simulink model "Offline_DataImport_AND_ECGAnalysis_AND_SCGAnalysis"  (R2020b)
settings: Solver=FixedStepDiscrete  StartTime=0.0  StopTime=param_sim_time  FixedStep=1/fs  MaxStep=1/fs  RelTol=1e-3
undefined symbols (not defined in the file): analyses, fdesignblkfcn, fs, gcbh, param_tot_samples
libraries: dspstat3 x1
(part 3 of 5)

== system Offline_DataImport_AND_ECGAnalysis_AND_SCGAnalysis/ECG Preprocessing/Enabled ECG Preprocessing Subsystem/ECG Filtfiltering/Bandpass Filter 2 ==
  In : Inport
  Generated Filter Block : DiscreteFir  Tag=BlockMethodSubSystem  Coefficients=[-0.0114243088354877773 0.00587624110456374388 0.00413946068324517157 0.00264334557424035672 0.00138774422276622192 0.00039597756815762733 -0.000357391963790950132 -0.000870027328167087902 -0.00118474210009046274 -0.0013114772414377189 -0.00130211118137258525 -0.00117028348293094116 -0.000969555288066135598 -0.000709991739662891794 -0.000441672338585462343 -0.000165596169411169614 7.38618239838010476e-05 0.000289182992126718261 0.00043918297873611449 0.000554539538172022298 0.000596791094711021305 0.000591852861038305242 0.000558642096174625374 0.000449318410474004379 0.000334719809825502479 0.00020575650819831294 5.39363215079843861e-05 -0.000101322531501510382 -0.000240833690149395291 -0.000354646039305753225 -0.000451018706232981029 -0.000523127741752206499 -0.000570171746042747937 -0.000579976289078059509 -0.000560050610609794802 -0.000510203484091005868 -0.000444253999700439106 -0.000361620699264023418 -0.000270418439597897714 -0.000171285996548194847 -6.96491449474114649e-05 2.51074882581126674e-05 0.000107701466472475207 0.000177443554931332875 0.000215288445749358542 0.000245848468855064048 0.000245696970898627229 0.000229649686627229205 0.00019096241212286473 0.000142984412950488554 7.04459950623022302e-05 -8.24128026295257998e-06 -9.80593727097200246e-05 -0.000181512369773678683 -0.000268731962362029828 -0.000342263684306691809 -0.000409113387221587271 -0.000453067377901137172 -0.000486836085121275519 -0.000497275928952340546 -0.00049828288783324709 -0.000472232231767717378 -0.00043821960462679492 -0.000378588991066479766 -0.000316844305738618603 -0.000241178452312015845 -0.000166037327502541535 -8.72939132895780845e-05 -1.92312446675550752e-05 4.72061762121969014e-05 9.32922079647201252e-05 0.000128677828260322091 0.000142225646220916352 0.000145392718308013161 0.000124316294889322346 9.22525950362868691e-05 3.91139366419743922e-05 -2.09540055264127723e-05 -9.84817072707550728e-05 -0.000176447200533612 -0.000261969930569216219 -0.000338398170707415388 -0.000413673787246831778 -0.000474956484152477126 -0.000526126847064748229 -0.000557031780194342657 -0.000573463759814568652 -0.000565518328802135789 -0.000545968260267525388 -0.000503292825521842527 -0.000450686144492560767 -0.00038193732270500047 -0.000310533512604118864 -0.000229221000311531989 -0.000153634622944792687 -7.7008709436998668e-05 -1.29951882972875049e-05 4.41972427699440645e-05 7.97744827227258452e-05 0.000101355022460052069 9.88614688825825011e-05 8.13696224336354218e-05 3.98982051577762009e-05 -1.42484593806998378e-05 -8.82654671942838254e-05 -0.000167074457359766074 -0.00025963077237387 -0.000347989994374806391 -0.000439444994547399936 -0.00051811479354047299 -0.000590082617058047473 -0.000641838802120880611 -0.000681503522967578934 -0.000694804478821137508 -0.00069209853970065606 -0.000663795693677639645 -0.000621757222242421206 -0.000557224399686986893 -0.000484587241980041772 -0.000396687438130890677 -0.000308737174406251494 -0.000214743893139471981 -0.00013218336614707546 -5.38482479860227792e-05 3.99111044497961476e-06 4.92154210607297082e-05 6.74354760492514721e-05 6.74472479585495194e-05 4.02217001782036176e-05 -4.06942016077313506e-06 -7.33562872444193381e-05 -0.000154074998390272069 -0.000252782754343081062 -0.000354062465090758047 -0.000462222943123069205 -0.000562271536985421011 -0.000658661832374597689 -0.000735808311790427799 -0.000799943578584080828 -0.000838241882526128551 -0.000857844739487072239 -0.000847533102258754556 -0.000817418121589637975 -0.000760200301916437102 -0.000687422833072246636 -0.000595027809558780832 -0.000496080524377292761 -0.000387710990138089018 -0.000284208196984854847 -0.000182518571703508756 -9.84384035011120345e-05 -2.73607674165961268e-05 1.77508990696524649e-05 4.21653277528823839e-05 3.53040248291924125e-05 5.59921773045889137e-06 -5.46825757556310132e-05 -0.000133739024050423885 -0.000236066993422962002 -0.000348549704079315764 -0.000473403235651745358 -0.000595572390038458938 -0.000716976323207035166 ...(+20655 chars)]  InputProcessing=Columns as channels (frame based)
  Out : Outport  VectorParamsAs1DForOutWhenUnconnected=off
  wires:
  Generated Filter Block/1 -> Out/1
  In/1 -> Generated Filter Block/1

== system Offline_DataImport_AND_ECGAnalysis_AND_SCGAnalysis/ECG Preprocessing/Enabled ECG Preprocessing Subsystem/To Workspace: Processed ECG/Enabled To Workspace ECG Subsystem ==
  note: The subsystem is only enabled when it receives a (non-zero) signal
  In1 : Inport
  Enable : EnablePort
  To Workspace ECG : ToWorkspace  VariableName=out_ecg_preprocessing  SaveFormat=Structure  SampleTime=-1
  wires:
  In1/1 -> To Workspace ECG/1

== system Offline_DataImport_AND_ECGAnalysis_AND_SCGAnalysis/SCG Analysis/Enabled SCG Analysis Subsystem/Anisotropy Characterization/Average Cycle Max Diameter//Volume Calculator ==
  in_r_pos : Inport
  in_scg_xyz : Inport  Port=2
  S1 Selector : Selector  NumberOfDimensions=2  InputPortWidth=3  IndexOptions=Index vector (dialog),Index vector (dialog)  Indices=[1:fs*0.2],[1 2 3]  OutputSizes=1,1
  SCG xyz Average Cycle : Subsystem
  Wrapped Average Cycle Max Diameter/Volume Calculator : MATLAB Function  TreatAsAtomicUnit=on
  out_average_cycle_max_diameter/volume : Outport
  wires:
  Wrapped Average Cycle Max Diameter/Volume Calculator/1(avg_cycle_max_diameter_over_volume) -> out_average_cycle_max_diameter/volume/1
  SCG xyz Average Cycle/1(out_scg_xyz_avgcycle) -> S1 Selector/1
  in_scg_xyz/1 -> SCG xyz Average Cycle/2(in_scg_xyz)
  in_r_pos/1 -> SCG xyz Average Cycle/1(in_ecg_r)
  S1 Selector/1 -> Wrapped Average Cycle Max Diameter/Volume Calculator/1(avg_s1_xyz)  "avg_scg_xyz_s1"

== system Offline_DataImport_AND_ECGAnalysis_AND_SCGAnalysis/SCG Analysis/Enabled SCG Analysis Subsystem/Anisotropy Characterization/Average Cycle Max//Median Diameter Calculator ==
  in_r_pos : Inport
  in_scg_xyz : Inport  Port=2
  S1 Selector : Selector  NumberOfDimensions=2  InputPortWidth=3  IndexOptions=Index vector (dialog),Index vector (dialog)  Indices=[1:fs*0.2],[1 2 3]  OutputSizes=1,1
  SCG xyz Average Cycle : Subsystem
  Wrapped Average Cycle Max/Median Diameter Calculator : MATLAB Function  TreatAsAtomicUnit=on
  out_average_cycle_max/median_diameter : Outport
  wires:
  Wrapped Average Cycle Max/Median Diameter Calculator/1(avg_cycle_max_over_median_diameter) -> out_average_cycle_max/median_diameter/1
  SCG xyz Average Cycle/1(out_scg_xyz_avgcycle) -> S1 Selector/1
  in_scg_xyz/1 -> SCG xyz Average Cycle/2(in_scg_xyz)
  in_r_pos/1 -> SCG xyz Average Cycle/1(in_ecg_r)
  S1 Selector/1 -> Wrapped Average Cycle Max/Median Diameter Calculator/1(avg_s1_xyz)  "avg_scg_xyz_s1"

== system Offline_DataImport_AND_ECGAnalysis_AND_SCGAnalysis/SCG Analysis/Enabled SCG Analysis Subsystem/Anisotropy Characterization/Average Cycle Max//Min Diameter Calculator ==
  in_r_pos : Inport
  in_scg_xyz : Inport  Port=2
  S1 Selector : Selector  NumberOfDimensions=2  InputPortWidth=3  IndexOptions=Index vector (dialog),Index vector (dialog)  Indices=[1:fs*0.2],[1 2 3]  OutputSizes=1,1
  SCG xyz Average Cycle : Subsystem
  Wrapped Average Cycle Max/Min Diameters Calculator : MATLAB Function  TreatAsAtomicUnit=on
  out_average_cycle_max/min_diameter : Outport
  wires:
  S1 Selector/1 -> Wrapped Average Cycle Max/Min Diameters Calculator/1(avg_s1_xyz)  "avg_scg_xyz_s1"
  in_r_pos/1 -> SCG xyz Average Cycle/1(in_ecg_r)
  in_scg_xyz/1 -> SCG xyz Average Cycle/2(in_scg_xyz)
  SCG xyz Average Cycle/1(out_scg_xyz_avgcycle) -> S1 Selector/1
  Wrapped Average Cycle Max/Min Diameters Calculator/1(avg_cycle_max_over_min_diameters) -> out_average_cycle_max/min_diameter/1

== system Offline_DataImport_AND_ECGAnalysis_AND_SCGAnalysis/SCG Analysis/Enabled SCG Analysis Subsystem/Anisotropy Characterization/Average Max Diameter//Volume Calculator ==
  in_r_pos : Inport
  in_scg_xyz : Inport  Port=2
  Constant1 : Constant  Value=fs
  Wrapped Average Max Diameter/Volume Calculator : MATLAB Function  TreatAsAtomicUnit=on
  out_average_max_diameter/volume : Outport
  wires:
  Constant1/1 -> Wrapped Average Max Diameter/Volume Calculator/1(fs)
  Wrapped Average Max Diameter/Volume Calculator/1(avg_max_diameter_over_volume) -> out_average_max_diameter/volume/1
  in_scg_xyz/1 -> Wrapped Average Max Diameter/Volume Calculator/3(scg_xyz)
  in_r_pos/1 -> Wrapped Average Max Diameter/Volume Calculator/2(r_pos)

== system Offline_DataImport_AND_ECGAnalysis_AND_SCGAnalysis/SCG Analysis/Enabled SCG Analysis Subsystem/Anisotropy Characterization/Average Max//Median Diameter Calculator ==
  in_r_pos : Inport
  in_scg_xyz : Inport  Port=2
  Constant1 : Constant  Value=fs
  Wrapped Average Max/Median Diameter Calculator : MATLAB Function  TreatAsAtomicUnit=on
  out_average_max/median_diameter : Outport
  wires:
  Constant1/1 -> Wrapped Average Max/Median Diameter Calculator/1(fs)
  Wrapped Average Max/Median Diameter Calculator/1(avg_max_over_median_diameter) -> out_average_max/median_diameter/1
  in_scg_xyz/1 -> Wrapped Average Max/Median Diameter Calculator/3(scg_xyz)
  in_r_pos/1 -> Wrapped Average Max/Median Diameter Calculator/2(r_pos)

== system Offline_DataImport_AND_ECGAnalysis_AND_SCGAnalysis/SCG Analysis/Enabled SCG Analysis Subsystem/Anisotropy Characterization/Average Max//Min Diameter Calculator ==
  in_r_pos : Inport
  in_scg_xyz : Inport  Port=2
  Constant1 : Constant  Value=fs
  Wrapped Average Max/Min Diameters Calculator : MATLAB Function  TreatAsAtomicUnit=on
  out_average_max/min_diameter : Outport
  wires:
  in_r_pos/1 -> Wrapped Average Max/Min Diameters Calculator/2(r_pos)
  in_scg_xyz/1 -> Wrapped Average Max/Min Diameters Calculator/3(scg_xyz)
  Wrapped Average Max/Min Diameters Calculator/1(avg_max_over_min_diameters) -> out_average_max/min_diameter/1
  Constant1/1 -> Wrapped Average Max/Min Diameters Calculator/1(fs)

== system Offline_DataImport_AND_ECGAnalysis_AND_SCGAnalysis/SCG Analysis/Enabled SCG Analysis Subsystem/Signal Generation/2D Mod Average Cycle ==
  in_r_pos : Inport
  in_2DMod : Inport  Port=2
  Average 2DMod Cycle Calculator : MATLAB Function  TreatAsAtomicUnit=on
  out_2DMod_avgcycle : Outport  VectorParamsAs1DForOutWhenUnconnected=off
  wires:
  in_r_pos/1 -> Average 2DMod Cycle Calculator/1(r_pos)
  in_2DMod/1 -> Average 2DMod Cycle Calculator/2(signal)
  Average 2DMod Cycle Calculator/1(avg_cycle) -> out_2DMod_avgcycle/1

== system Offline_DataImport_AND_ECGAnalysis_AND_SCGAnalysis/SCG Analysis/Enabled SCG Analysis Subsystem/Signal Generation/2DMod Calculator ==
  in_scg_xyz : Inport
  2DMod Calculator : Subsystem
  Constant : Constant  Value=xyz2Dcombo
  Multiport Switch : MultiPortSwitch
  xy Selector : Selector  NumberOfDimensions=2  IndexOptions=Select all,Index vector (dialog)  Indices=[1:min(analyses.ecg.RR)],[1 2]  OutputSizes=1,1
  xz Selector2 : Selector  NumberOfDimensions=2  IndexOptions=Select all,Index vector (dialog)  Indices=[1:min(analyses.ecg.RR)],[1 3]  OutputSizes=1,1
  yz Selector1 : Selector  NumberOfDimensions=2  IndexOptions=Select all,Index vector (dialog)  Indices=[1:min(analyses.ecg.RR)],[2 3]  OutputSizes=1,1
  out_2DMod : Outport  VectorParamsAs1DForOutWhenUnconnected=off
  wires:
  2DMod Calculator/1(2D Modulus) -> out_2DMod/1
  in_scg_xyz/1 -> xz Selector2/1, xy Selector/1, yz Selector1/1
  Constant/1 -> Multiport Switch/1
  Multiport Switch/1 -> 2DMod Calculator/1(2D Components)
  xy Selector/1 -> Multiport Switch/2
  yz Selector1/1 -> Multiport Switch/3
  xz Selector2/1 -> Multiport Switch/4

== system Offline_DataImport_AND_ECGAnalysis_AND_SCGAnalysis/SCG Analysis/Enabled SCG Analysis Subsystem/Signal Generation/3D Mod Average Cycle ==
  in_r_pos : Inport
  in_3DMod : Inport  Port=2
  Average 3DMod Cycle Calculator : MATLAB Function  TreatAsAtomicUnit=on
  out_3DMod_avgcycle : Outport  VectorParamsAs1DForOutWhenUnconnected=off
  wires:
  Average 3DMod Cycle Calculator/1(avg_cycle) -> out_3DMod_avgcycle/1
  in_3DMod/1 -> Average 3DMod Cycle Calculator/2(signal)
  in_r_pos/1 -> Average 3DMod Cycle Calculator/1(r_pos)

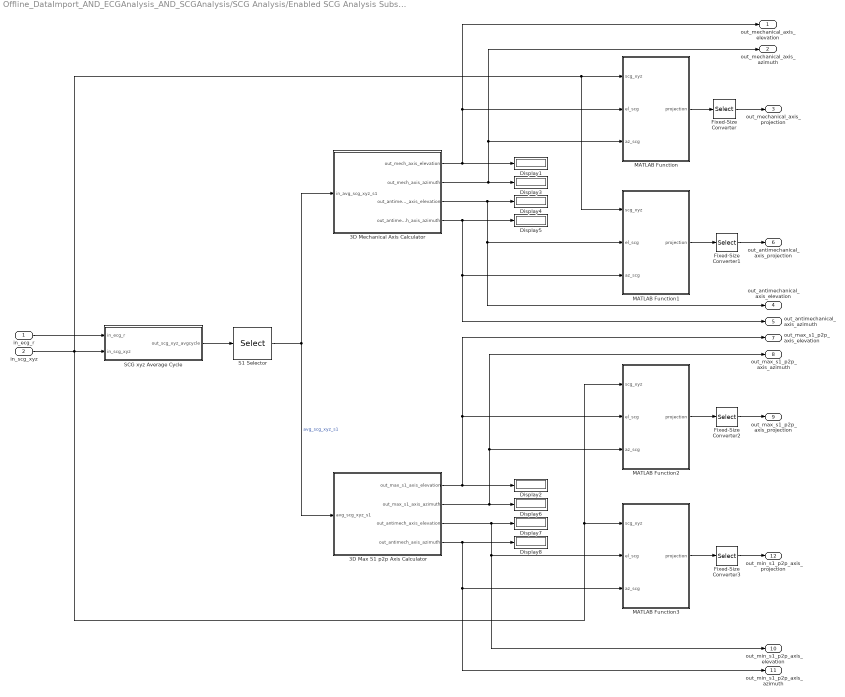
== system Offline_DataImport_AND_ECGAnalysis_AND_SCGAnalysis/SCG Analysis/Enabled SCG Analysis Subsystem/Signal Generation/3D Projections ==
  in_ecg_r : Inport
  in_scg_xyz : Inport  Port=2
  3D Max S1 p2p Axis Calculator : Subsystem
  3D Mechanical Axis Calculator : Subsystem
  Display{1..8} (8 alike) : Display
  Fixed-Size Converter{,1..3} (4 alike) : Selector  NumberOfDimensions=2  IndexOptions=Index vector (dialog),Index vector (dialog)  Indices=[1:param_tot_samples],[1]  OutputSizes=1,1
  MATLAB Function : MATLAB Function  TreatAsAtomicUnit=on
  MATLAB Function1 : MATLAB Function  TreatAsAtomicUnit=on
  MATLAB Function2 : MATLAB Function  TreatAsAtomicUnit=on
  MATLAB Function3 : MATLAB Function  TreatAsAtomicUnit=on
  S1 Selector : Selector  NumberOfDimensions=2  InputPortWidth=3  IndexOptions=Index vector (dialog),Index vector (dialog)  Indices=[1:fs*0.2],[1 2 3]  OutputSizes=1,1
  SCG xyz Average Cycle : Subsystem
  out_mechanical_axis_elevation : Outport
  out_mechanical_axis_azimuth : Outport  Port=2
  out_mechanical_axis_projection : Outport  Port=3
  out_antimechanical_axis_elevation : Outport  Port=4
  out_antimechanical_axis_azimuth : Outport  Port=5
  out_antimechanical_axis_projection : Outport  Port=6
  out_max_s1_p2p_axis_elevation : Outport  Port=7
  out_max_s1_p2p_axis_azimuth : Outport  Port=8
  out_max_s1_p2p_axis_projection : Outport  Port=9
  out_min_s1_p2p_axis_elevation : Outport  Port=10
  out_min_s1_p2p_axis_azimuth : Outport  Port=11
  out_min_s1_p2p_axis_projection : Outport  Port=12
  wires:
  in_scg_xyz/1 -> SCG xyz Average Cycle/2(in_scg_xyz), MATLAB Function/1(scg_xyz), MATLAB Function1/1(scg_xyz), MATLAB Function2/1(scg_xyz), MATLAB Function3/1(scg_xyz)
  S1 Selector/1 -> 3D Max S1 p2p Axis Calculator/1(avg_scg_xyz_s1), 3D Mechanical Axis Calculator/1(in_avg_scg_xyz_s1)  "avg_scg_xyz_s1"
  SCG xyz Average Cycle/1(out_scg_xyz_avgcycle) -> S1 Selector/1
  MATLAB Function2/1(projection) -> Fixed-Size Converter2/1
  MATLAB Function1/1(projection) -> Fixed-Size Converter1/1
  MATLAB Function/1(projection) -> Fixed-Size Converter/1
  Fixed-Size Converter/1 -> out_mechanical_axis_projection/1
  Fixed-Size Converter1/1 -> out_antimechanical_axis_projection/1
  Fixed-Size Converter2/1 -> out_max_s1_p2p_axis_projection/1
  MATLAB Function3/1(projection) -> Fixed-Size Converter3/1
  Fixed-Size Converter3/1 -> out_min_s1_p2p_axis_projection/1
  3D Mechanical Axis Calculator/2(out_mech_axis_azimuth) -> Display3/1, out_mechanical_axis_azimuth/1, MATLAB Function/3(az_scg)
  3D Mechanical Axis Calculator/3(out_antimech_axis_elevation) -> Display4/1, out_antimechanical_axis_elevation/1, MATLAB Function1/2(el_scg)
  3D Mechanical Axis Calculator/1(out_mech_axis_elevation) -> Display1/1, out_mechanical_axis_elevation/1, MATLAB Function/2(el_scg)
  3D Mechanical Axis Calculator/4(out_antimech_axis_azimuth) -> Display5/1, out_antimechanical_axis_azimuth/1, MATLAB Function1/3(az_scg)
  3D Max S1 p2p Axis Calculator/4(out_antimech_axis_azimuth) -> Display8/1, out_min_s1_p2p_axis_azimuth/1, MATLAB Function3/3(az_scg)
  3D Max S1 p2p Axis Calculator/2(out_max_s1_axis_azimuth) -> out_max_s1_p2p_axis_azimuth/1, MATLAB Function2/3(az_scg), Display6/1
  3D Max S1 p2p Axis Calculator/3(out_antimech_axis_elevation) -> out_min_s1_p2p_axis_elevation/1, MATLAB Function3/2(el_scg), Display7/1
  3D Max S1 p2p Axis Calculator/1(out_max_s1_axis_elevation) -> out_max_s1_p2p_axis_elevation/1, MATLAB Function2/2(el_scg), Display2/1
  in_ecg_r/1 -> SCG xyz Average Cycle/1(in_ecg_r)

== system Offline_DataImport_AND_ECGAnalysis_AND_SCGAnalysis/SCG Analysis/Enabled SCG Analysis Subsystem/Signal Generation/3DMod Calculator ==
  in_scgxyz : Inport
  Square Root1 : Sqrt  SaturateOnIntegerOverflow=on
  Square1 : Math  Operator=square  SignedPower=on  SaturateOnIntegerOverflow=on
  Sum1 : Sum  Inputs=+  CollapseMode=Specified dimension  CollapseDim=2
  out_3DMod : Outport  VectorParamsAs1DForOutWhenUnconnected=off
  wires:
  Square1/1 -> Sum1/1
  Sum1/1 -> Square Root1/1
  in_scgxyz/1 -> Square1/1
  Square Root1/1 -> out_3DMod/1
